simulink model "last_example_at_section"  (R2021a)
settings: Solver=VariableStepAuto  StartTime=0.0  StopTime=10  MaxStep=1e-3  RelTol=1e-3
libraries: simulink x1
settings Model: Creator=YasserNet  LastModifiedBy=YasserNet

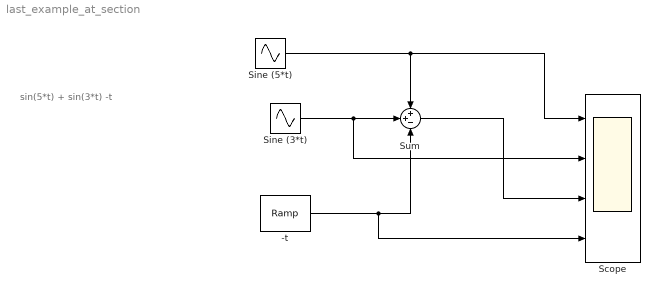
== system last_example_at_section ==
  note: sin(5*t) + sin(3*t) -t
  -t : simulink/Sources/Ramp  slope=1  start=0  InitialOutput=0
  Scope : Scope  NumInputPorts=4
  Sine (3*t) : Sin  Phase=3  SampleTime=0
  Sine (5*t) : Sin  Frequency=5  SampleTime=0
  Sum : Sum  Inputs=++-
  wires:
  Sine (3*t)/1 -> Sum/2, Scope/2
  Sine (5*t)/1 -> Sum/1, Scope/1
  -t/1 -> Sum/3, Scope/4
  Sum/1 -> Scope/3
